simulink model "MSICA_Projet1_StructureModaleSansControle"  (R2018a)
settings: Solver=VariableStepAuto  StartTime=0.0  StopTime=10.0  RelTol=1e-3
values from neighbouring files (symbols this model uses):
  A_S1_S2 = [ zeros(3,3) eye(3) ... (first row only)    [DonneesProjet.m]
  Amod = [zeros(3) eye(3); -omega_carre -2*xi*sqrt(omega_carre)]    [DonneesProjet.m]
  B_S1_S2 = [zeros(3,3); inv(M_S1_S2)]    [DonneesProjet.m]
  Bmod = [zeros(3); phi']    [DonneesProjet.m]
  C1 = [eye(3) zeros(3,3)]    [DonneesProjet.m]
  Cmod = [phi zeros(3,3)]    [DonneesProjet.m]
settings Model: Creator=natha  LastModifiedBy=natha
settings DataIOCC: ReturnWorkspaceOutputs=on
settings SFSimCC: SimUseLocalCustomCode=on
settings RTWCC: RTWUseLocalCustomCode=on

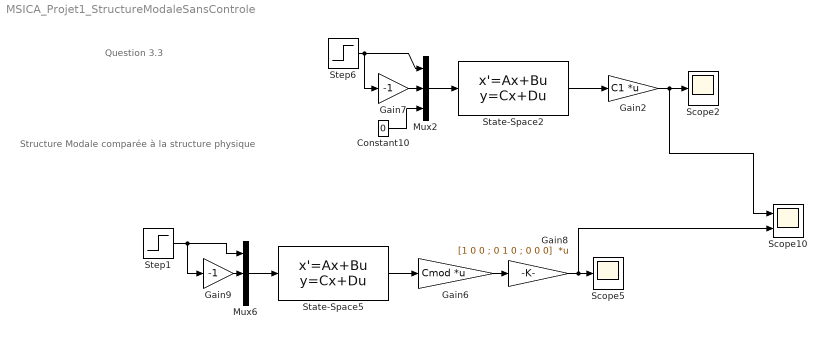
== system MSICA_Projet1_StructureModaleSansControle ==
  note: Structure Modale comparée à la structure physique
  note: Question 3.3
  Constant10 : Constant  Value=0
  Gain2 : Gain  Gain=C1  Multiplication=Matrix(K*u)
  Gain6 : Gain  Gain=Cmod  Multiplication=Matrix(K*u)
  Gain7 : Gain  Gain=-1
  Gain8 : Gain  Gain=[1 0 0 ; 0 1 0 ; 0 0 0]  Multiplication=Matrix(K*u)
  Gain9 : Gain  Gain=-1
  Mux2 : Mux  Inputs=3
  Mux6 : Mux  Inputs=3
  Scope10 : Scope  NumInputPorts=2
  Scope2 : Scope
  Scope5 : Scope
  State-Space2 : StateSpace  A=A_S1_S2  B=B_S1_S2  C=eye(6)  D=zeros(6,3)  InitialCondition=0
  State-Space5 : StateSpace  A=Amod  B=Bmod  C=eye(6)  D=zeros(6,3)  InitialCondition=0
  Step1 : Step  Time=0.001  Before=100  After=0  SampleTime=0
  Step6 : Step  Time=0.001  Before=100  After=0  SampleTime=0
  wires:
  State-Space2/1 -> Gain2/1
  Mux2/1 -> State-Space2/1
  Step6/1 -> Mux2/1, Gain7/1
  Constant10/1 -> Mux2/3
  Gain7/1 -> Mux2/2
  Gain2/1 -> Scope10/1, Scope2/1
  Gain6/1 -> Gain8/1
  Mux6/1 -> State-Space5/1
  Step1/1 -> Gain9/1, Mux6/1
  Gain9/1 -> Mux6/2
  Gain8/1 -> Scope10/2, Scope5/1
  State-Space5/1 -> Gain6/1
